simulink model "quad_simulink_wPosition"  (R2013a)
settings: Solver=ode3  StartTime=0.0  StopTime=30  FixedStep=0.05  MaxStep=.1  RelTol=1e-3
model workspace (MAT data in the model file):
  Sig = Simulink.Signal
  Sig.DataType = 'auto'
  Sig.Dimensions = -1
  Sig.DimensionsMode = 'auto'
  Sig.Complexity = 'auto'
  Sig.SampleTime = -1
  Sig.SamplingMode = 'auto'
values from neighbouring files (symbols this model uses):
  quadModel = struct('g',(g),'d',(d),'mass',(mass),'ct',(ct),'cq',(cq),'Jx',(Jx),'Jy',(Jy),'Jz',(Jz),'Jb',(Jb),'Jbinv',(Jbinv),'dctcq',(dctcq),     'motor_m',(motor_m),'motor_dm',(motor_dm),'motor_h',(motor_h),'motor_r',(motor_r),     'ESC_m',(ESC_m),'ESC_a',(ESC_a),'ESC_b',(ESC_b),'ESC_ds',(ESC_ds),     'HUB_m',(HUB_m),'HUB_r',(HUB_r),'HUB_L',(HUB_L),     'arms_m',(arms_m),'arms_r',(arms_r),'arms_L',(arms_L),' ...(+48 chars)    [GUI_1.m]
undefined symbols (not defined in the file or in its folder): IC
libraries: simulink x4
settings Model: Creator=Kevin  LastModifiedBy=Kevin
settings Model: ModifiedComment=|
  | davidhartman -- Sun Feb 23 01:41:19 2014 -- Version 1.71
  | + Added experimental saturation to the attitude controller
settings Model: ModifiedHistory=|
  | davidhartman -- Sun Feb 23 01:41:19 2014 -- Version 1.71
  | + Added experimental saturation to the attitude controller
  | 
  | davidhartman -- Sun Feb 23 00:43:12 2014 -- Version 1.70
  | + Added derivative term to the XY position controller. Seems to improve response and allow for higher propertional gains though the pitch angles are sometimes more aggressive
  | + Further improvements to both XY and attitude controller gains
  | + Numerous description changes and labeling improvements
  | + Added lots of color to the main view and resized and repositioned the buttons to try to create a more useful layout.
  | 
  | TO DO:
  | ~ Add saturation to position controller output
  | ~ Improve plotting functions: add desired position to state data plot and creat a GUI for the Flight animation
  | 
  | davidhartman -- Sat Feb 22 21:53:07 2014 -- Version 1.69
  | + Cleaned up a bit, nothing major
  | 
  | davidhartman -- Sat Feb 22 21:07:22 2014 -- Version 1.68
  | + Created substystems for position and altitude control and improved yaw, and XY gains.
  | + Added a simin from workspace input to allow for timeseries position data to be imported from the workspace...still experimental
  | 
  | davidhartman -- Sat Feb 22 19:23:03 2014 -- Version 1.67
  | + Rough Control of X-Y
  | 
  | TO DO
  | ~ Clean up the mess, seperate atitude and XY control aspects
  | ~ Tune for better performance (use damping term? Integral?)
  | ~ Still need to add disturbances to model
  | 
  | davidhartman -- Sat Feb 22 18:18:27 2014 -- Version 1.66
  | +lol matlab is crashing and making me save
  | 
  | davidhartman -- Sat Feb 22 16:50:46 2014 -- Version 1.65
  | + changed the way the derivative term is calculated for theta, still need to do phi, theta.
  | 
  | davidhartman -- Sat Feb 22 15:25:37 2014 -- Version 1.64
  | + First attempt towards X-Y control
  | 
  | davidhartman -- Sat Feb 22 14:26:16 2014 -- Version 1.63
  | + Fixed motor IC's to scale properly
  | + Adjusted motor control mixing and Psi control gains
  | 
  | davidhartman -- Sat Feb 22 00:06:15 2014 -- Version 1.62
  | + Rough implementation of Phi, Theta, and Psi control
  | + No other major changes,
  | 
  | Kevin -- Tue Feb 18 21:50:16 2014 -- Version 1.60
  | + Organized buttons on left of diagram
  | + Added 2 buttons: 1st is to open the main GUI, 2nd is to open the IC's GUI
  | 
  | davidhartman -- Sun Feb 16 14:17:49 2014 -- Version 1.59
  | 
  | 
  | davidhartman -- Sun Feb 16 13:52:55 2014 -- Version 1.58
  | + killed off feedback for pitch/roll/yaw for now
  | 
  | davidhartman -- Sun Feb 16 13:22:45 2014 -- Version 1.57
  | NUMEROUS IMPORTANT CHANGES:
  | +Added system sim start check to see if quadModel and ICs are loaded, puts out message block...could be better but works.
  | +changed quad structure name to quadModel to stop having errors related to the MATLAB built in function "quad()"
  | +Updated calls to quadModel within the simulation to use the right name
  | +added cr and b to the quadModel .mat file ("Team37quad.mat")
  | +Fixed the Altitude control...this required doing some basic math to find the required motor speed for gravity cancelation as a function of measured parameters (now including ct and b). This means the Z control now works infinitely better than before since it doesnt saturate the motors. The reason roll and pitch didn't work is because the Z correction term was insanely large..In the future we might want to try adding individual saturations to each control term (Z, Phi, The, Psi) so that none of them can individually overload the motor signal..
  | +Updated yout to include motor commands for plotting post simulation
  | +Added motor commands to QuadPlotForSimulink script and converted the units in the script to ft.
  | 
  | TO DO:
  | ~Add cr and b to the GUI
  | ~Fix controllers for Phi,The,Psi to at least sort of work
  | ~Fix units on animation function
  | ~Add disturbance inputs to S-function (tauPhi-The-Psi, Fx-y-z) for disturbance rejection testing
  | ~Add sensor simulation block or something
  | ~X-Y controller
  | 
  | KEVIN:
  | +Help me make a GUI for the quad plot animation. You know a lot more about GUI's than me at this point so I need help
  | 
  | Kevin -- Thu Feb 13 18:17:20 2014 -- Version 1.54
  | + Fixed labels on buttons to left
  | + Motor dynamic states blocks: now pull IC's from IC structure... also the A parameter is fixed to show +/- 1/T where T is time constant (saved in quad.mat)
  | + S function file updated to newest file "...v06_SI" - still not ready as far as unit conversions go
  | + Added IC as a parameter to the S func options
  | 
  | davidhartman -- Thu Feb 13 05:04:45 2014 -- Version 1.53
  | + fixed the motor dynamics block to properly apply the RPM gains in cooperation with the throttle cuttof (important since we aren't forcing a zero intercept fit...)
  | + added some coments, particularly concerning the motor command mixing, which will need to change if we change our coordinate axis.
  | TO DO:
  | Unchanged from last save, and:
  | ~Decide whether to change coordinate axis to the full-blown stndard aircraft configuration (see Corke book or aircraft dynamics book/lectures)
  | 
  | davidhartman -- Wed Feb 12 18:15:18 2014 -- Version 1.52
  | + Deleted a commented out stop script
  | 
  | davidhartman -- Wed Feb 12 18:08:27 2014 -- Version 1.51
  | + numerous updates,including a new S-function that has been checked for correct SI unit logic.
  | + Small ducumentation updates
  | + Small change or two to plotting buttons
  | TO DO:
  | ~ Same as last save for the most part
  | ~ Finish units conversion for GUI's and related spots (Kevin took notes)
  | ~ IC's structure, options structure....?, etc.
  | ~ Fix controllers...is it okay to use Phi/Theta/Psi? how about PQR?
  | ~ dun dun dun...cost functions and optimiztion script...
  | 
  | davidhartman -- Wed Feb 12 01:31:21 2014 -- Version 1.50
  | + updated the scaling for the motors to be more complete
  | + added saturation to motors
  | + added w^2 to S function
  | +started looking into units (They are still not right...grrr.)
  | +added throttle cutoff
  | +changed buttons to be smarter and cooler
  | +worried about things that might be wrong with this thing,,,
  | TO DO:
  | It's getting pretty complex already...before adding to much more complexity:
  | ~Nail down units. No Excuses.
  | ~Go through state equations and verify they are correct and reasonably efficient, eliminating junk code
  | ~Maybe start thinking about improving the controllers to be more reasonable...maybe repeat your rough controller approximation using a rough model and MATLAB
  | 
  | Kevin -- Sun Feb 09 12:27:21 2014 -- Version 1.46
  | + Added 2 custom function blocks to left of Simulation diagram
  | + Block 1 brings up standard load window to load desired structure
  | + Block 2 runs the animation file --- must run the Simulation first
  | 
  | Kevin -- Sun Feb 09 12:16:15 2014 -- Version 1.45
  | +
  | 
  | Kevin -- Sun Feb 09 10:30:33 2014 -- Version 1.44
  | + aVal should = 1/T ... we were using aVal = T
  | 
  | Kevin -- Sat Feb 08 13:05:40 2014 -- Version 1.43
  | + Under "Model Properties --> InitFcn" --- changed to uiload instead of load('quad.mat') --- (this required that every structure must be named quad.mat)
  | 
  | + A load window is now displayed so you can select which structure to load into the Simulink
  | 
  | Kevin -- Fri Feb 07 10:12:57 2014 -- Version 1.42
  | + Updated the a parameter to quad.aVal --- from the quad structure (GUI)
  | + Updated the w IC's to quad.wIC --- from the quad structure (GUI)
  | 
  | davidhartman -- Wed Feb 05 16:39:32 2014 -- Version 1.41
  | + Updated s-function to use quad model values from parameter input on mask
  | + cleaned up from past efforts
  | TO DO:
  | + add w1_IC and a values to quad structure
  | + add GUI buttons
  | 
  | davidhartman -- Wed Feb 05 13:06:04 2014 -- Version 1.40
  | + changed motor dynamics to state space form to allow ic's to be set (w1_ic, etc.)
  | + packaged motor dynamics into a block
  | + made small adjustments to state equation block...unsucceful at improving data import of "quad.mat" structure...this still needs work.
  | + some color coding experimentation
  | + parameterization of time constant for motors (a = 1/T), and ic's.
  | + small changes to model space comments
  | TO DO:
  | ~ Create a block library for project?
  | 
  | davidhartman -- Tue Jan 28 21:08:29 2014 -- Version 1.38
  | +added unit gain motor delays for now
  | +trial and error improved PID values
  | +changed a few small simulation settings on recomendation of "model advisor"
  | +added several scopes to ease troubleshooting
  | +working on improving naming and documentation within the simulink models
  | 
  | davidhartman -- Tue Jan 28 12:00:35 2014 -- Version 1.37
  | +fixed some residual motor control issues...still more to do.
  | +added motor speeds to state output
  | 
  | davidhartman -- Tue Jan 28 11:37:54 2014 -- Version 1.36
  | +fixed denominator of PD control gains to match fall term ode function
  | +fixed motor control equations and tidied things up
  | +adjustments to inti function, loading the quad.mat variables differently...still needs work.
settings DataIOCC: LimitDataPoints=off  SignalLogging=off
settings OptimizationCC: InlineParams=on
settings DebuggingCC: UniqueDataStoreMsg=warning  StrictBusMsg=WarnOnBusTreatedAsVector

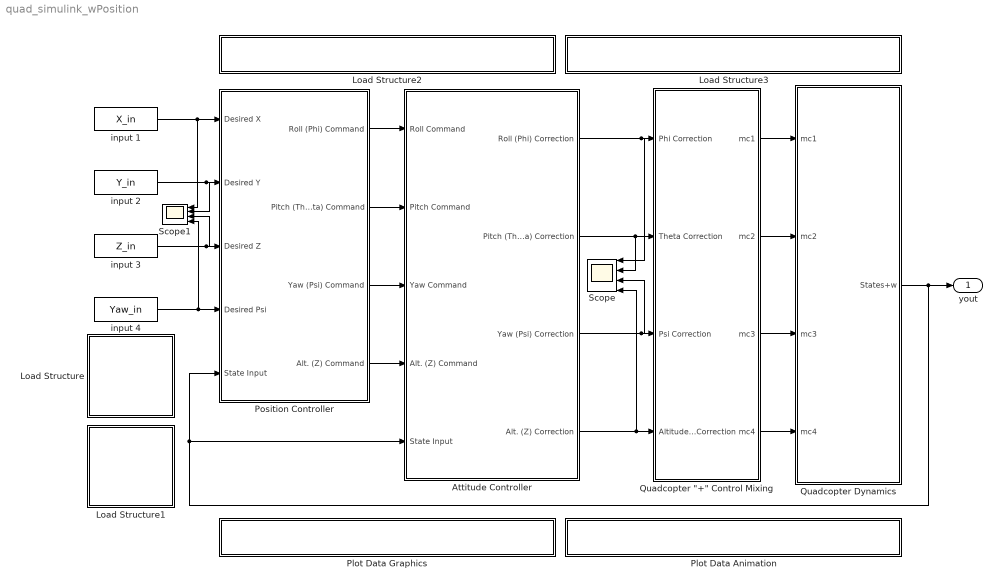
== system quad_simulink_wPosition ==
  Attitude Controller : Subsystem
  Load Structure : Subsystem
      settings: OpenFcn=uiload
      mask Display: fprintf('LOAD:\nQuadcopter\nModel');
  Load Structure1 : Subsystem
      settings: OpenFcn=uiload
      mask Display: fprintf('LOAD:\nInitial\nConditions')
  Load Structure2 : Subsystem
      settings: OpenFcn=|
      | if exist('GUI_1') == 2,
      | run('GUI_1')
      | 
      | else
      | 
      | msgbox('The desired GUI must be first added to MATLABs path.')
      | 
      | end
      mask Display: fprintf('OPEN GUI: Build New \n Model');
  Load Structure3 : Subsystem
      settings: OpenFcn=|
      | if exist('GUI_IC') == 2,
      | run('GUI_IC')
      | 
      | else
      | 
      | msgbox('The desired GUI must be first added to MATLABs path.')
      | 
      | end
      mask Display: fprintf('OPEN GUI: Create Initial \n Conditions');
  Plot Data Animation : Subsystem
      settings: OpenFcn=|
      | if exist('QuadAnim') == 2,
      | run('QuadAnim')
      | 
      | else
      | 
      | msgbox('The desired GUI must be first added to MATLABs path.')
      | 
      | end
      mask Display: fprintf('OPEN PLOT: Flight Animation')
  Plot Data Graphics : Subsystem
      settings: OpenFcn=|
      | if exist('yout')
      | Quad_plot_forsimulink
      | else
      | msgbox('Simulation must be run before data can be plotted.')
      | end
      mask Display: fprintf('OPEN PLOT: State Data')
  Position Controller : Subsystem
  "Quadcopter \"+\" Control Mixing" : Subsystem
  Quadcopter Dynamics : Subsystem
  Scope : Scope  NumInputPorts=4
      settings: YMin=-5~-5~-5~-5  YMax=5~5~5~5  SaveName=ScopeData5
  Scope1 : Scope  NumInputPorts=4
      settings: YMin=-5~-5~-5~-5  YMax=5~5~5~5  SaveName=ScopeData7
  input 1 : FromWorkspace  VariableName=X_in  SampleTime=0  Interpolate=off  OutputAfterFinalValue=Holding final value
  input 2 : FromWorkspace  VariableName=Y_in  SampleTime=0  Interpolate=off  OutputAfterFinalValue=Holding final value
  input 3 : FromWorkspace  VariableName=Z_in  SampleTime=0  Interpolate=off  OutputAfterFinalValue=Holding final value
  input 4 : FromWorkspace  VariableName=Yaw_in  SampleTime=0  Interpolate=off  OutputAfterFinalValue=Holding final value
  yout : Outport
  wires:
  Quadcopter Dynamics/1(States+w) -> yout/1, Attitude Controller/5(State Input), Position Controller/5(State Input)
  "Quadcopter \"+\" Control Mixing"/1(mc1) -> Quadcopter Dynamics/1(mc1)
  "Quadcopter \"+\" Control Mixing"/2(mc2) -> Quadcopter Dynamics/2(mc2)
  "Quadcopter \"+\" Control Mixing"/3(mc3) -> Quadcopter Dynamics/3(mc3)
  "Quadcopter \"+\" Control Mixing"/4(mc4) -> Quadcopter Dynamics/4(mc4)
  Attitude Controller/1(Roll (Phi) Correction) -> Scope/1, "Quadcopter \"+\" Control Mixing"/1(Phi Correction)
  Attitude Controller/3(Yaw (Psi) Correction) -> Scope/3, "Quadcopter \"+\" Control Mixing"/3(Psi Correction)
  Attitude Controller/2(Pitch (Theta) Correction) -> "Quadcopter \"+\" Control Mixing"/2(Theta Correction), Scope/2
  Attitude Controller/4(Alt. (Z) Correction) -> "Quadcopter \"+\" Control Mixing"/4(Altitude Correction), Scope/4
  Position Controller/1(Roll (Phi) Command) -> Attitude Controller/1(Roll Command)
  Position Controller/2(Pitch (Theta) Command) -> Attitude Controller/2(Pitch Command)
  Position Controller/4(Alt. (Z) Command) -> Attitude Controller/4(Alt. (Z) Command)
  Position Controller/3(Yaw (Psi) Command) -> Attitude Controller/3(Yaw Command)
  input 1/1 -> Scope1/1, Position Controller/1(Desired X)
  input 4/1 -> Scope1/4, Position Controller/4(Desired Psi)
  input 3/1 -> Scope1/3, Position Controller/3(Desired Z)
  input 2/1 -> Scope1/2, Position Controller/2(Desired Y)

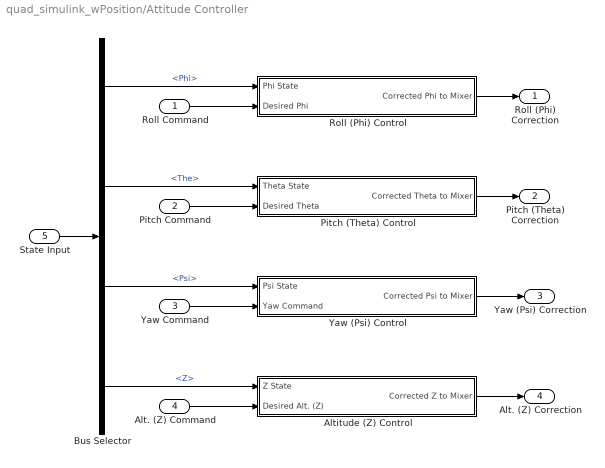
== system quad_simulink_wPosition/Attitude Controller ==
  Roll Command : Inport
  Pitch Command : Inport  Port=2
  Yaw Command : Inport  Port=3
  Alt. (Z) Command : Inport  Port=4
  State Input : Inport  Port=5
  Altitude (Z) Control : Subsystem
      mask Display:
      | port_label('input',1,'Z State')
      | port_label('output',1,'Corrected Z')
  Bus Selector : BusSelector  OutputSignals=Phi,The,Psi,Z
  Pitch (Theta) Control : Subsystem
      mask Display:
      | port_label('input',1,'Theta State')
      | port_label('output',1,'Corrected Theta')
  "Roll (Phi) Control " : Subsystem
      mask Display:
      | port_label('input',1,'Phi State')
      | port_label('output',1,'Corrected Phi')
  Yaw (Psi) Control : Subsystem
      mask Display:
      | port_label('input',1,'Psi State')
      | port_label('output',1,'Corrected Psi')
  Roll (Phi) Correction : Outport
  Pitch (Theta) Correction : Outport  Port=2
  Yaw (Psi) Correction : Outport  Port=3
  Alt. (Z) Correction : Outport  Port=4
  wires:
  Altitude (Z) Control/1(Corrected Z to Mixer) -> Alt. (Z) Correction/1
  Yaw (Psi) Control/1(Corrected Psi to Mixer) -> Yaw (Psi) Correction/1
  Pitch (Theta) Control/1(Corrected Theta to Mixer) -> Pitch (Theta) Correction/1
  "Roll (Phi) Control "/1(Corrected Phi to Mixer) -> Roll (Phi) Correction/1
  Bus Selector/4 -> Altitude (Z) Control/1(Z State)  "<Z>"
  Bus Selector/3 -> Yaw (Psi) Control/1(Psi State)  "<Psi>"
  Bus Selector/1 -> "Roll (Phi) Control "/1(Phi State)  "<Phi>"
  Bus Selector/2 -> Pitch (Theta) Control/1(Theta State)  "<The>"
  State Input/1 -> Bus Selector/1
  Roll Command/1 -> "Roll (Phi) Control "/2(Desired Phi)
  Pitch Command/1 -> Pitch (Theta) Control/2(Desired Theta)
  Alt. (Z) Command/1 -> Altitude (Z) Control/2(Desired Alt. (Z))
  Yaw Command/1 -> Yaw (Psi) Control/2(Yaw Command)

== system quad_simulink_wPosition/Load Structure ==

== system quad_simulink_wPosition/Load Structure1 ==

== system quad_simulink_wPosition/Load Structure2 ==

== system quad_simulink_wPosition/Load Structure3 ==

== system quad_simulink_wPosition/Plot Data Animation ==

== system quad_simulink_wPosition/Plot Data Graphics ==

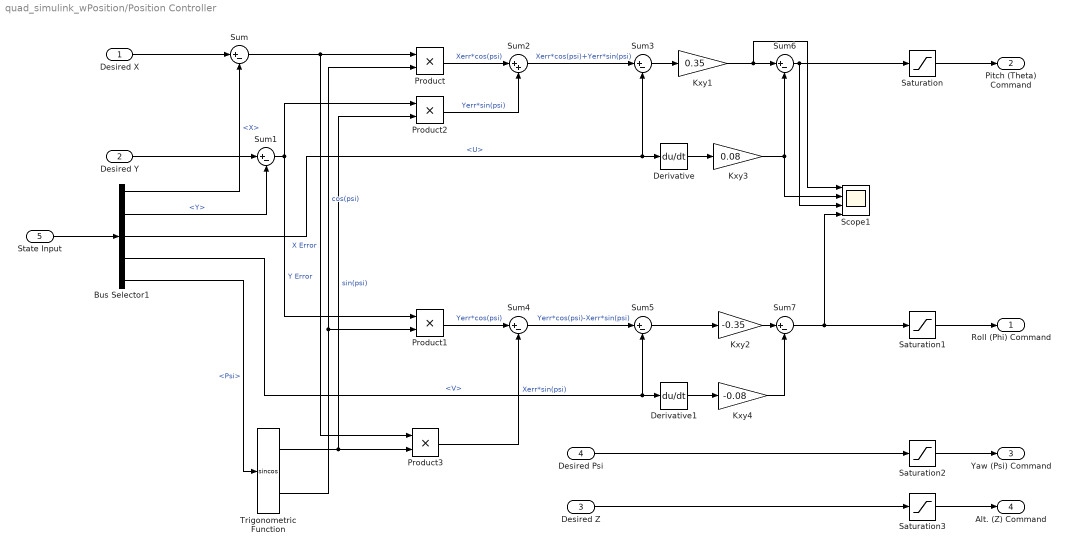
== system quad_simulink_wPosition/Position Controller ==
  Desired X : Inport
  Desired Y : Inport  Port=2
  Desired Z : Inport  Port=3
  Desired Psi : Inport  Port=4
  State Input : Inport  Port=5
  Bus Selector1 : BusSelector  OutputSignals=X,Y,U,V,Psi
  Derivative : Derivative
  Derivative1 : Derivative
  Kxy1 : Gain  Gain=0.35
  Kxy2 : Gain  Gain=-0.35
  Kxy3 : Gain  Gain=0.08
  Kxy4 : Gain  Gain=-0.08
  Product{,1..3} (4 alike) : Product
  Saturation{,1..3} (4 alike) : Saturate  UpperLimit=0.2  LowerLimit=-0.2
  Scope1 : Scope  NumInputPorts=4
      settings: ShowLegends=on  YMin=-5~-5~-5~-5  YMax=5~5~5~5  SaveName=ScopeData8
  Sum{,1,3..7} (7 alike) : Sum  Inputs=|+-
  Sum2 : Sum  Inputs=|++
  Trigonometric Function : Trigonometry  Operator=sincos
  Roll (Phi) Command : Outport
  Pitch (Theta) Command : Outport  Port=2
  Yaw (Psi) Command : Outport  Port=3
  Alt. (Z) Command : Outport  Port=4
  wires:
  Sum4/1 -> Sum5/1  "Yerr*cos(psi)-Xerr*sin(psi)"
  Bus Selector1/4 -> Derivative1/1, Sum5/2  "<V>"
  Sum5/1 -> Kxy2/1
  State Input/1 -> Bus Selector1/1
  Product2/1 -> Sum2/2  "Yerr*sin(psi)"
  Product1/1 -> Sum4/1  "Yerr*cos(psi)"
  Product3/1 -> Sum4/2  "Xerr*sin(psi)"
  Sum1/1 -> Product2/1, Product1/1  "Y Error"
  Sum2/1 -> Sum3/1  "Xerr*cos(psi)+Yerr*sin(psi)"
  Sum3/1 -> Kxy1/1
  Bus Selector1/3 -> Derivative/1, Sum3/2  "<U>"
  Desired Z/1 -> Saturation3/1
  Bus Selector1/5 -> Trigonometric Function/1  "<Psi>"
  Desired X/1 -> Sum/1
  Bus Selector1/1 -> Sum/2  "<X>"
  Desired Y/1 -> Sum1/1
  Bus Selector1/2 -> Sum1/2  "<Y>"
  Sum/1 -> Product3/1, Product/1  "X Error"
  Trigonometric Function/2 -> Product/2, Product1/2  "cos(psi)"
  Product/1 -> Sum2/1  "Xerr*cos(psi)"
  Trigonometric Function/1 -> Product2/2, Product3/2  "sin(psi)"
  Desired Psi/1 -> Saturation2/1
  Kxy1/1 -> Scope1/1, Sum6/1
  Sum6/1 -> Scope1/3, Saturation/1
  Kxy3/1 -> Sum6/2, Scope1/2
  Derivative/1 -> Kxy3/1
  Derivative1/1 -> Kxy4/1
  Kxy2/1 -> Sum7/1
  Sum7/1 -> Scope1/4, Saturation1/1
  Kxy4/1 -> Sum7/2
  Saturation/1 -> Pitch (Theta) Command/1
  Saturation1/1 -> Roll (Phi) Command/1
  Saturation2/1 -> Yaw (Psi) Command/1
  Saturation3/1 -> Alt. (Z) Command/1

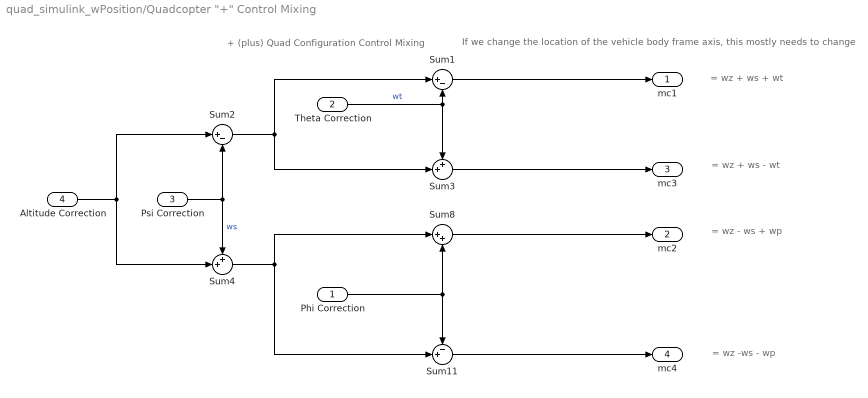
== system quad_simulink_wPosition/Quadcopter "+" Control Mixing ==
  note: If we change the location of the vehicle body frame axis, this mostly needs to change
  note: = wz + ws + wt
  note: + (plus) Quad Configuration Control Mixing
  note: = wz + ws - wt
  note: = wz - ws + wp
  note: = wz -ws - wp
  Phi Correction : Inport
  Theta Correction : Inport  Port=2
  Psi Correction : Inport  Port=3
  Altitude Correction : Inport  Port=4
  Sum1 : Sum  Inputs=|+-
  Sum11 : Sum  Inputs=-+|
  Sum2 : Sum  Inputs=|+-
  Sum3 : Sum  Inputs=++|
  Sum4 : Sum  Inputs=++|
  Sum8 : Sum  Inputs=|++
  mc1 : Outport
  mc2 : Outport  Port=2
  mc3 : Outport  Port=3
  mc4 : Outport  Port=4
  wires:
  Theta Correction/1 -> Sum3/1, Sum1/2  "wt"
  Altitude Correction/1 -> Sum2/1, Sum4/2
  Sum2/1 -> Sum3/2, Sum1/1
  Psi Correction/1 -> Sum4/1, Sum2/2  "ws"
  Sum4/1 -> Sum11/2, Sum8/1
  Sum8/1 -> mc2/1
  Sum11/1 -> mc4/1
  Phi Correction/1 -> Sum8/2, Sum11/1
  Sum3/1 -> mc3/1
  Sum1/1 -> mc1/1

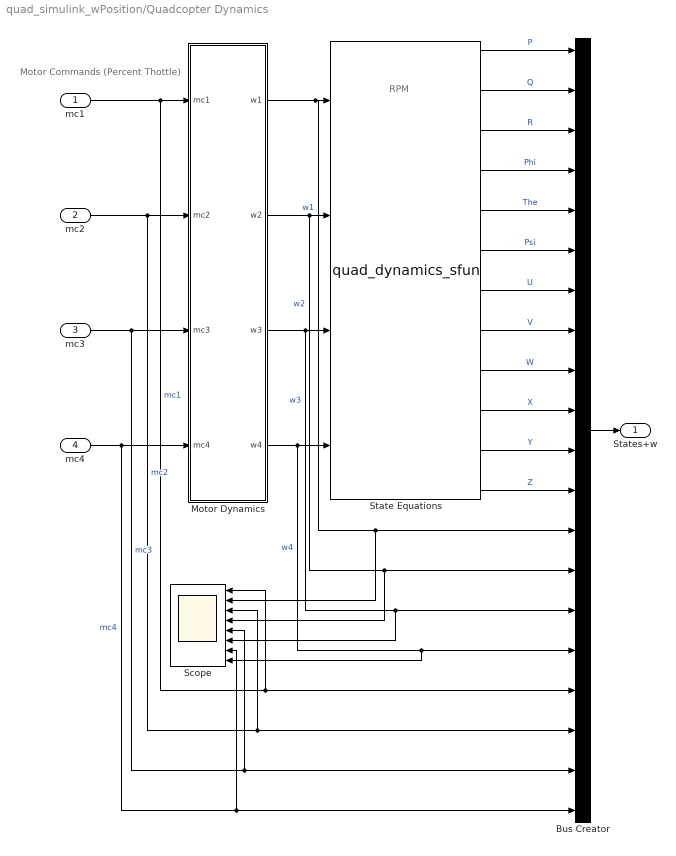
== system quad_simulink_wPosition/Quadcopter Dynamics ==
  note: RPM
  note: Motor Commands
      | (Percent Thottle)
  mc1 : Inport
  mc2 : Inport  Port=2
  mc3 : Inport  Port=3
  mc4 : Inport  Port=4
  Bus Creator : BusCreator  Inputs='P','Q','R','Phi','The','Psi','U','V','W','X','Y','Z','w1','w2','w3','w4','mc1','mc2','mc3','mc4'
  Motor Dynamics : Subsystem
  Scope : Scope  NumInputPorts=8
      settings: YMin=-5~-5~-5~-5~-5~-5~-5~-5  YMax=5~5~5~5~5~5~5~5  SaveName=ScopeData4
  State Equations : M-S-Function  FunctionName=quad_dynamics_sfun  Parameters=quadModel, IC
  States+w : Outport
  wires:
  mc1/1 -> Scope/1, Bus Creator/17, Motor Dynamics/1(mc1)  "mc1"
  mc2/1 -> Scope/3, Bus Creator/18, Motor Dynamics/2(mc2)  "mc2"
  mc3/1 -> Motor Dynamics/3(mc3), Scope/5, Bus Creator/19  "mc3"
  mc4/1 -> Motor Dynamics/4(mc4), Scope/7, Bus Creator/20  "mc4"
  State Equations/1 -> Bus Creator/1  "P"
  State Equations/2 -> Bus Creator/2  "Q"
  State Equations/3 -> Bus Creator/3  "R"
  State Equations/4 -> Bus Creator/4  "Phi"
  State Equations/5 -> Bus Creator/5  "The"
  State Equations/6 -> Bus Creator/6  "Psi"
  State Equations/7 -> Bus Creator/7  "U"
  State Equations/8 -> Bus Creator/8  "V"
  State Equations/9 -> Bus Creator/9  "W"
  State Equations/10 -> Bus Creator/10  "X"
  State Equations/11 -> Bus Creator/11  "Y"
  State Equations/12 -> Bus Creator/12  "Z"
  Bus Creator/1 -> States+w/1
  Motor Dynamics/1(w1) -> Scope/2, Bus Creator/13, State Equations/1  "w1"
  Motor Dynamics/2(w2) -> State Equations/2, Scope/4, Bus Creator/14  "w2"
  Motor Dynamics/3(w3) -> State Equations/3, Scope/6, Bus Creator/15  "w3"
  Motor Dynamics/4(w4) -> Scope/8, Bus Creator/16, State Equations/4  "w4"

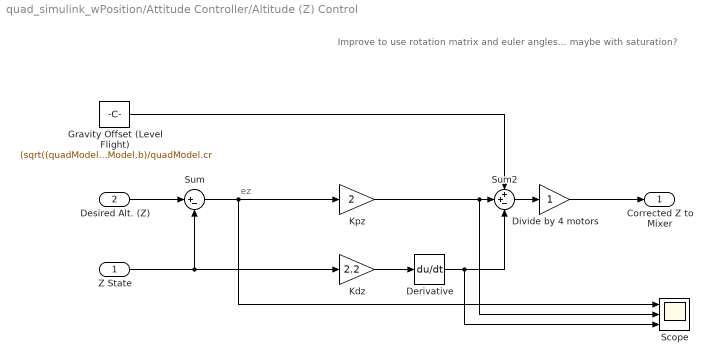
== system quad_simulink_wPosition/Attitude Controller/Altitude (Z) Control ==
  note: Improve to use rotation matrix and euler angles...
      | maybe with saturation?
  note: ez
  Z State : Inport
  Desired Alt. (Z) : Inport  Port=2
  Derivative : Derivative
  Divide by 4 motors : Gain
  Gravity Offset (Level Flight) : Constant  Value=(sqrt((quadModel.mass*quadModel.g)/(4*quadModel.ct))-quadModel.b)/quadModel.cr
  Kdz : Gain  Gain=2.2
  Kpz : Gain  Gain=2
  Scope : Scope  NumInputPorts=3
      settings: YMin=-5~-5~-5  YMax=5~5~5
  Sum : Sum  Inputs=|+-
  Sum2 : Sum  Inputs=++-
  Corrected Z to Mixer : Outport
  wires:
  Gravity Offset (Level Flight)/1 -> Sum2/1
  Sum/1 -> Scope/1, Kpz/1
  Kdz/1 -> Derivative/1
  Desired Alt. (Z)/1 -> Sum/1
  Z State/1 -> Kdz/1, Sum/2
  Derivative/1 -> Scope/3, Sum2/3
  Sum2/1 -> Divide by 4 motors/1
  Divide by 4 motors/1 -> Corrected Z to Mixer/1
  Kpz/1 -> Scope/2, Sum2/2

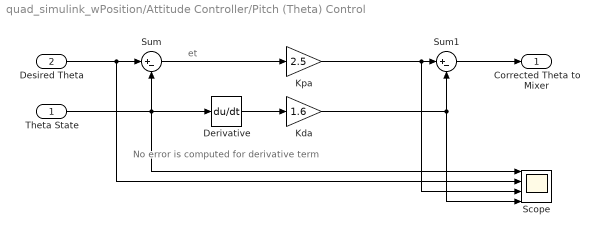
== system quad_simulink_wPosition/Attitude Controller/Pitch (Theta) Control ==
  note: No error is computed for
      | derivative term
  note: et
  Theta State : Inport
  Desired Theta : Inport  Port=2
  Derivative : Derivative
  Kda : Gain  Gain=1.6
  Kpa : Gain  Gain=2.5
  Scope : Scope  NumInputPorts=4
      settings: YMin=-5~-5~-5~-5  YMax=5~5~5~5  SaveName=ScopeData3
  Sum : Sum  Inputs=|+-
  Sum1 : Sum  Inputs=|+-
  Corrected Theta to Mixer : Outport
  wires:
  Sum/1 -> Kpa/1
  Desired Theta/1 -> Scope/2, Sum/1
  Sum1/1 -> Corrected Theta to Mixer/1
  Theta State/1 -> Scope/1, Derivative/1, Sum/2
  Kda/1 -> Scope/4, Sum1/2
  Kpa/1 -> Scope/3, Sum1/1
  Derivative/1 -> Kda/1

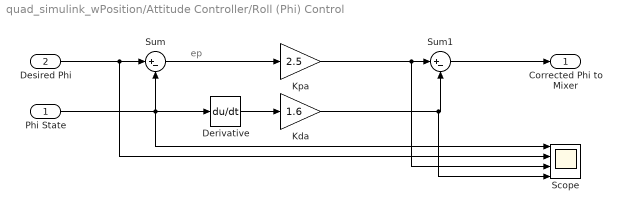
== system quad_simulink_wPosition/Attitude Controller/Roll (Phi) Control  ==
  note: ep
  Phi State : Inport
  Desired Phi : Inport  Port=2
  Derivative : Derivative
  Kda : Gain  Gain=1.6
  Kpa : Gain  Gain=2.5
  Scope : Scope  NumInputPorts=4
      settings: YMin=-5~-5~-5~-5  YMax=5~5~5~5
  Sum : Sum  Inputs=|+-
  Sum1 : Sum  Inputs=|+-
  Corrected Phi to Mixer : Outport
  wires:
  Sum/1 -> Kpa/1
  Desired Phi/1 -> Scope/2, Sum/1
  Phi State/1 -> Scope/1, Derivative/1, Sum/2
  Sum1/1 -> Corrected Phi to Mixer/1
  Kpa/1 -> Scope/3, Sum1/1
  Derivative/1 -> Kda/1
  Kda/1 -> Scope/4, Sum1/2

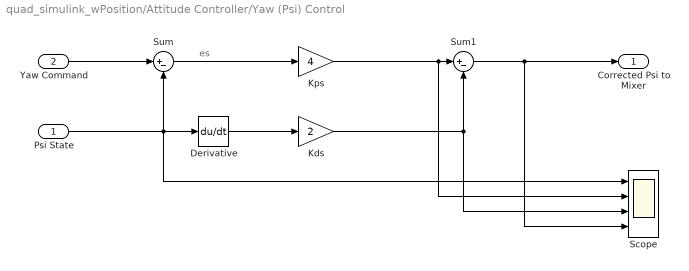
== system quad_simulink_wPosition/Attitude Controller/Yaw (Psi) Control ==
  note: es
  Psi State : Inport
  Yaw Command : Inport  Port=2
  Derivative : Derivative
  Kds : Gain  Gain=2
  Kps : Gain  Gain=4
  Scope : Scope  NumInputPorts=4
      settings: YMin=-5~-5~-5~-5  YMax=5~5~5~5  SaveName=ScopeData2
  Sum : Sum  Inputs=|+-
  Sum1 : Sum  Inputs=|+-
  Corrected Psi to Mixer : Outport
  wires:
  Sum/1 -> Kps/1
  Yaw Command/1 -> Sum/1
  Sum1/1 -> Scope/4, Corrected Psi to Mixer/1
  Psi State/1 -> Derivative/1, Scope/1, Sum/2
  Kps/1 -> Scope/2, Sum1/1
  Derivative/1 -> Kds/1
  Kds/1 -> Scope/3, Sum1/2

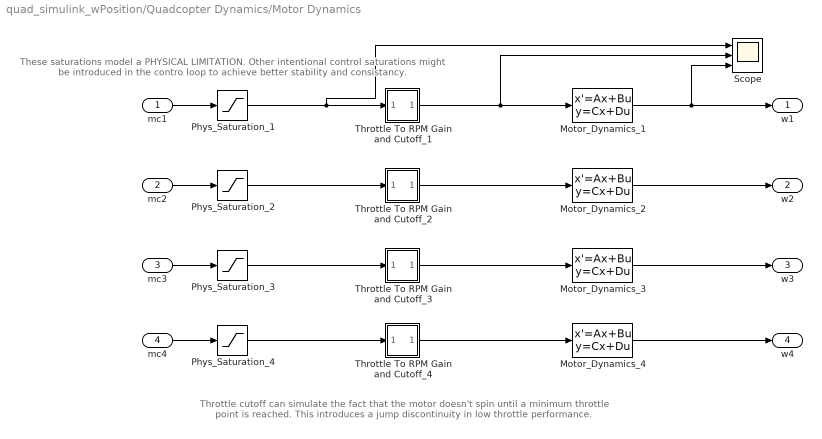
== system quad_simulink_wPosition/Quadcopter Dynamics/Motor Dynamics ==
  note: Throttle cutoff can simulate the fact that the motor doesn't
      | spin until a minimum throttle point is reached. This introduces
      | a jump discontinuity in low throttle performance.
  note: These saturations model a PHYSICAL LIMITATION.
      | Other intentional control saturations might be introduced in the
      | contro loop to achieve better stability and consistancy.
  mc1 : Inport
  mc2 : Inport  Port=2
  mc3 : Inport  Port=3
  mc4 : Inport  Port=4
  Motor_Dynamics_1 : StateSpace  A=-1/quadModel.T  C=1/quadModel.T  D=0  X0=IC.w1*quadModel.T
  Motor_Dynamics_2 : StateSpace  A=-1/quadModel.T  C=1/quadModel.T  D=0  X0=IC.w2*quadModel.T
  Motor_Dynamics_3 : StateSpace  A=-1/quadModel.T  C=1/quadModel.T  D=0  X0=IC.w3*quadModel.T
  Motor_Dynamics_4 : StateSpace  A=-1/quadModel.T  C=1/quadModel.T  D=0  X0=IC.w4*quadModel.T
  Phys_Saturation_{1..4} (4 alike) : Saturate  UpperLimit=100  LowerLimit=0
  Scope : Scope  NumInputPorts=3
      settings: ShowLegends=on  YMin=-5~-5~-5  YMax=5~5~5  SaveName=ScopeData6
  Throttle To RPM Gain and Cutoff_1 : Subsystem
  Throttle To RPM Gain and Cutoff_2 : Subsystem
  Throttle To RPM Gain and Cutoff_3 : Subsystem
  Throttle To RPM Gain and Cutoff_4 : Subsystem
  w1 : Outport
  w2 : Outport  Port=2
  w3 : Outport  Port=3
  w4 : Outport  Port=4
  wires:
  mc1/1 -> Phys_Saturation_1/1
  mc4/1 -> Phys_Saturation_4/1
  mc2/1 -> Phys_Saturation_2/1
  mc3/1 -> Phys_Saturation_3/1
  Phys_Saturation_1/1 -> Scope/1, Throttle To RPM Gain and Cutoff_1/1(In5)
  Phys_Saturation_2/1 -> Throttle To RPM Gain and Cutoff_2/1(In5)
  Phys_Saturation_3/1 -> Throttle To RPM Gain and Cutoff_3/1(In5)
  Phys_Saturation_4/1 -> Throttle To RPM Gain and Cutoff_4/1(In5)
  Throttle To RPM Gain and Cutoff_1/1(Out5) -> Scope/2, Motor_Dynamics_1/1
  Throttle To RPM Gain and Cutoff_2/1(Out5) -> Motor_Dynamics_2/1
  Throttle To RPM Gain and Cutoff_3/1(Out5) -> Motor_Dynamics_3/1
  Throttle To RPM Gain and Cutoff_4/1(Out5) -> Motor_Dynamics_4/1
  Motor_Dynamics_1/1 -> Scope/3, w1/1
  Motor_Dynamics_2/1 -> w2/1
  Motor_Dynamics_3/1 -> w3/1
  Motor_Dynamics_4/1 -> w4/1

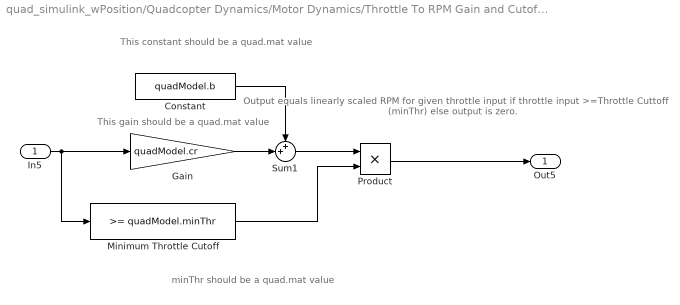
== system quad_simulink_wPosition/Quadcopter Dynamics/Motor Dynamics/Throttle To RPM Gain and Cutoff_1 ==
  note: minThr should be a quad.mat value
  note: This gain should be a quad.mat value
  note: This constant should be a quad.mat value
  note: Output equals linearly scaled RPM
      | for given throttle input if throttle input >=Throttle Cuttoff (minThr)
      | else output is zero.
  In5 : Inport
  Constant : Constant  Value=quadModel.b
  Gain : Gain  Gain=quadModel.cr
  Minimum Throttle Cutoff : simulink/Logic and Bit Operations/Compare To Constant  relop=>=  const=quadModel.minThr  OutDataTypeStr=uint8
  Product : Product
  Sum1 : Sum  Inputs=++|
  Out5 : Outport
  wires:
  Minimum Throttle Cutoff/1 -> Product/2
  Product/1 -> Out5/1
  In5/1 -> Gain/1, Minimum Throttle Cutoff/1
  Gain/1 -> Sum1/2
  Sum1/1 -> Product/1
  Constant/1 -> Sum1/1

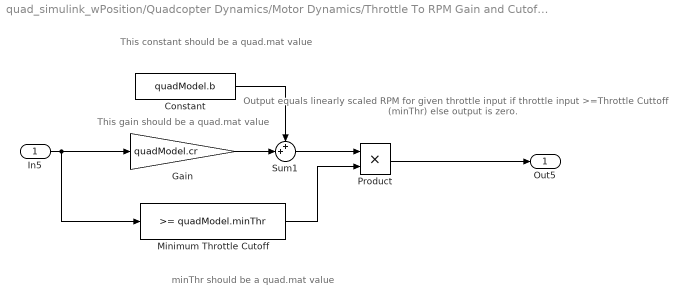
== system quad_simulink_wPosition/Quadcopter Dynamics/Motor Dynamics/Throttle To RPM Gain and Cutoff_2 ==
  note: minThr should be a quad.mat value
  note: This gain should be a quad.mat value
  note: This constant should be a quad.mat value
  note: Output equals linearly scaled RPM
      | for given throttle input if throttle input >=Throttle Cuttoff (minThr)
      | else output is zero.
  In5 : Inport
  Constant : Constant  Value=quadModel.b
  Gain : Gain  Gain=quadModel.cr
  Minimum Throttle Cutoff : simulink/Logic and Bit Operations/Compare To Constant  relop=>=  const=quadModel.minThr  OutDataTypeStr=uint8
  Product : Product
  Sum1 : Sum  Inputs=++|
  Out5 : Outport
  wires:
  Minimum Throttle Cutoff/1 -> Product/2
  Product/1 -> Out5/1
  In5/1 -> Gain/1, Minimum Throttle Cutoff/1
  Gain/1 -> Sum1/2
  Sum1/1 -> Product/1
  Constant/1 -> Sum1/1

== system quad_simulink_wPosition/Quadcopter Dynamics/Motor Dynamics/Throttle To RPM Gain and Cutoff_3 ==
  note: minThr should be a quad.mat value
  note: This gain should be a quad.mat value
  note: This constant should be a quad.mat value
  note: Output equals linearly scaled RPM
      | for given throttle input if throttle input >=Throttle Cuttoff (minThr)
      | else output is zero.
  In5 : Inport
  Constant : Constant  Value=quadModel.b
  Gain : Gain  Gain=quadModel.cr
  Minimum Throttle Cutoff : simulink/Logic and Bit Operations/Compare To Constant  relop=>=  const=quadModel.minThr  OutDataTypeStr=uint8
  Product : Product
  Sum1 : Sum  Inputs=++|
  Out5 : Outport
  wires:
  Minimum Throttle Cutoff/1 -> Product/2
  Product/1 -> Out5/1
  In5/1 -> Gain/1, Minimum Throttle Cutoff/1
  Gain/1 -> Sum1/2
  Sum1/1 -> Product/1
  Constant/1 -> Sum1/1

== system quad_simulink_wPosition/Quadcopter Dynamics/Motor Dynamics/Throttle To RPM Gain and Cutoff_4 ==
  note: minThr should be a quad.mat value
  note: This gain should be a quad.mat value
  note: This constant should be a quad.mat value
  note: Output equals linearly scaled RPM
      | for given throttle input if throttle input >=Throttle Cuttoff (minThr)
      | else output is zero.
  In5 : Inport
  Constant : Constant  Value=quadModel.b
  Gain : Gain  Gain=quadModel.cr
  Minimum Throttle Cutoff : simulink/Logic and Bit Operations/Compare To Constant  relop=>=  const=quadModel.minThr  OutDataTypeStr=uint8
  Product : Product
  Sum1 : Sum  Inputs=++|
  Out5 : Outport
  wires:
  Minimum Throttle Cutoff/1 -> Product/2
  Product/1 -> Out5/1
  In5/1 -> Gain/1, Minimum Throttle Cutoff/1
  Gain/1 -> Sum1/2
  Sum1/1 -> Product/1
  Constant/1 -> Sum1/1
